simulink model "BatteryModel"  (R2019b)
settings: Solver=FixedStepAuto  StartTime=t(1)  StopTime=t(end)  FixedStep=0.005  RelTol=1e-3
values from neighbouring files (symbols this model uses):
  Temp_in = 46.327347    [input.mat]
libraries: fl_lib x1, nesl_utility x1
settings Model: Creator=PcElettronicaDynamis  LastModifiedBy=PcElettronicaDynamis
settings DataIOCC: SaveOutput=off  SignalLogging=off  DSMLogging=off  ReturnWorkspaceOutputsName=Sim

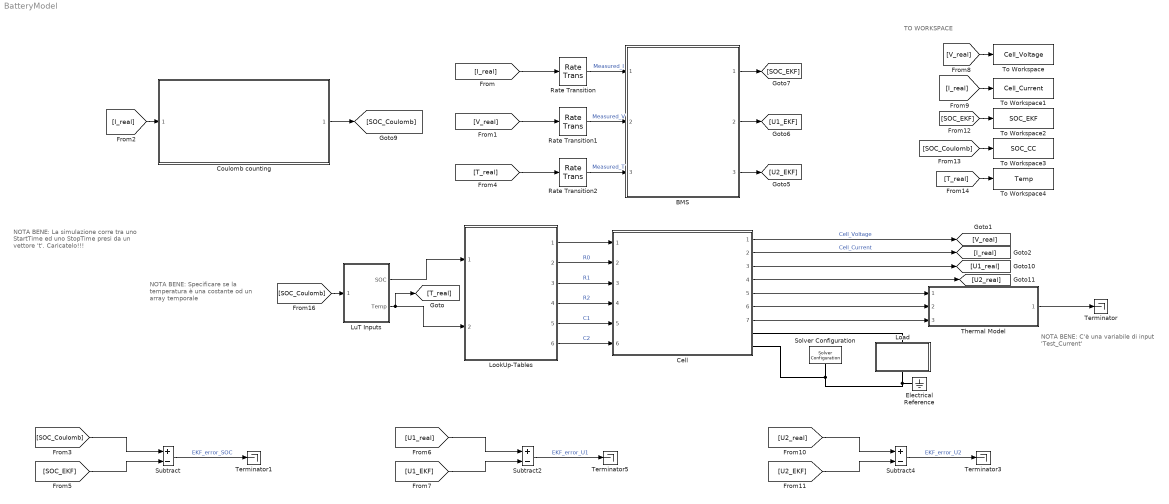
== system BatteryModel ==
  note: TO WORKSPACE
  note: NOTA BENE: La simulazione corre tra uno StartTime ed uno StopTime presi da un vettore 't'. Caricatelo!!!
  note: NOTA BENE: C'è una variabile di input 'Test_Current'
  note: NOTA BENE: Specificare se la temperatura è una costante od un array temporale
  BMS : Subsystem  ReferencedSubsystem=BMS
  Cell : Subsystem  ReferencedSubsystem=Cell
  Coulomb counting : Subsystem  ReferencedSubsystem=Coulomb_counting
  Electrical Reference : fl_lib/Electrical/Electrical Elements/Electrical Reference
  Load : Subsystem  ReferencedSubsystem=Load
  LookUp-Tables : Subsystem  ReferencedSubsystem=LuT
  LuT Inputs : Subsystem
  Rate Transition : RateTransition  OutPortSampleTime=0.005
  Rate Transition1 : RateTransition  OutPortSampleTime=0.005
  Rate Transition2 : RateTransition  OutPortSampleTime=0.005
  Solver Configuration : nesl_utility/Solver Configuration  PhysicalDomain=network_engine_domain  SubClassName=solver  LeftPortType=input  RightPortType=generic  Tones=[]  Harmonics=[]  SimulateNoise=off  Profile=off  UseLocalSampling=off  EnableSwitchedLinearOptims=on  FrequencyDomain=off  UseCCode=off  RelTol=0.001  AbsTol=1e-06  MinStep=1e-09  ToWorkspace=off  RevertToSquareIcSolve=off  NumHomotopyIterations=100  PhasorMode=off  PhasorModeNumHarmonics=1  DoDC=off  ResidualTolerance=1e-09  UseLocalSolver=off  LocalSolverChoice=NE_BACKWARD_EULER_ADVANCER  LocalSolverSampleTime=0.001  DoFixedCost=off  MaxNonlinIter=3  MaxModeIter=2  LinearAlgebra=auto  EquationFormulation=NE_TIME_EF  DelaysMemoryBudget=1024  AutomaticFiltering=on  FilteringTimeConstant=0.001  PartitionStorageMethod=AS_NEEDED  PartitionMemoryBudget=1024  PartitionMethod=ROBUST
  Subtract : Sum  Inputs=+-
  Subtract2 : Sum  Inputs=+-
  Subtract4 : Sum  Inputs=+-
  Terminator{,1,3,5} (4 alike) : Terminator
  Thermal Model : Subsystem  ReferencedSubsystem=ThermalModel
  To Workspace : ToWorkspace  VariableName=Cell_Voltage  SaveFormat=Timeseries  SampleTime=0.005
  To Workspace1 : ToWorkspace  VariableName=Cell_Current  SaveFormat=Timeseries  SampleTime=0.005
  To Workspace2 : ToWorkspace  VariableName=SOC_EKF  SaveFormat=Timeseries  SampleTime=0.005
  To Workspace3 : ToWorkspace  VariableName=SOC_CC  SaveFormat=Timeseries  SampleTime=0.005
  To Workspace4 : ToWorkspace  VariableName=Temp  SaveFormat=Timeseries  SampleTime=0.005
  wires:
  Cell/5 -> Thermal Model/1
  Cell/6 -> Thermal Model/2
  Cell/7 -> Thermal Model/3
  Coulomb counting/1 -> [SOC_Coulomb]
  LookUp-Tables/1 -> Cell/1
  LookUp-Tables/2 -> Cell/2  "R0"
  LookUp-Tables/3 -> Cell/3  "R1"
  LookUp-Tables/4 -> Cell/4  "R2"
  LookUp-Tables/5 -> Cell/5  "C1"
  LookUp-Tables/6 -> Cell/6  "C2"
  Cell/4 -> [U2_real]
  Cell/3 -> [U1_real]
  Cell/2 -> [I_real]  "Cell_Current"
  Cell/1 -> [V_real]  "Cell_Voltage"
  [V_real] -> Rate Transition1/1
  [T_real] -> Rate Transition2/1
  Rate Transition1/1 -> BMS/2  "Measured_V"
  [I_real] -> Rate Transition/1
  Rate Transition/1 -> BMS/1  "Measured_I"
  Rate Transition2/1 -> BMS/3  "Measured_T"
  [I_real] -> Coulomb counting/1
  [U1_real] -> Subtract2/1
  [U2_real] -> Subtract4/1
  [U1_EKF] -> Subtract2/2
  [SOC_Coulomb] -> Subtract/1
  Subtract4/1 -> Terminator3/1  "EKF_error_U2"
  Subtract/1 -> Terminator1/1  "EKF_error_SOC"
  [SOC_EKF] -> Subtract/2
  Subtract2/1 -> Terminator5/1  "EKF_error_U1"
  [U2_EKF] -> Subtract4/2
  BMS/1 -> [SOC_EKF]
  BMS/2 -> [U1_EKF]
  BMS/3 -> [U2_EKF]
  Thermal Model/1 -> Terminator/1
  [V_real] -> To Workspace/1
  [I_real] -> To Workspace1/1
  [SOC_EKF] -> To Workspace2/1
  [SOC_Coulomb] -> To Workspace3/1
  [T_real] -> To Workspace4/1
  LuT Inputs/1(SOC) -> LookUp-Tables/1
  LuT Inputs/2(Temp) -> [T_real], LookUp-Tables/2
  [SOC_Coulomb] -> LuT Inputs/1(SOC_CC)
  connections:
  Load/LConn1 -- Cell/RConn1
  Load/RConn1 -- Solver Configuration/RConn1 -- Cell/RConn2 -- Electrical Reference/LConn1

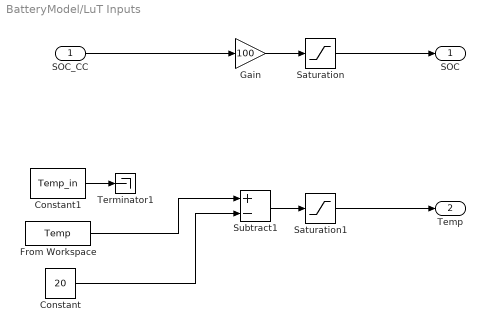
== system BatteryModel/LuT Inputs ==
  SOC_CC : Inport
  Constant : Constant  Value=20
  Constant1 : Constant  Value=Temp_in
  From Workspace : FromWorkspace  VariableName=Temp  SampleTime=0
  Gain : Gain  Gain=100
  Saturation : Saturate  UpperLimit=100  LowerLimit=1
  Saturation1 : Saturate  UpperLimit=40  LowerLimit=1
  Subtract1 : Sum  Inputs=+-
  Terminator1 : Terminator
  SOC : Outport
  Temp : Outport  Port=2
  wires:
  Saturation1/1 -> Temp/1
  Constant1/1 -> Terminator1/1
  From Workspace/1 -> Subtract1/1
  Saturation/1 -> SOC/1
  Gain/1 -> Saturation/1
  Constant/1 -> Subtract1/2
  Subtract1/1 -> Saturation1/1
  SOC_CC/1 -> Gain/1
